simulink model "IEEE_39_case2"  (R2024b)
settings: Solver=ode3  StartTime=0  StopTime=40  FixedStep=Ts  MaxStep=1/60  RelTol=1e-3  AbsTol=1e-3  EnableMultiTasking=on
values from neighbouring files (symbols this model uses):
  c_f = c_f*Cb    [fun00_GFL_pu_2_normial.m]    (also in fun00_GFM_pu_2_normial.m)
  Dt = 0    [s02_case1.m]    (also in s02_case2.m; s03_case3.m; s03_case4.m; s03_case5.m)
  dw0_sm = 0    [s02_case1.m]    (also in s02_case2.m; s03_case3.m; s03_case4.m; s03_case5.m)
  Emax = 1.3    [s02_case1.m]    (also in s02_case2.m; s03_case3.m; s03_case4.m; s03_case5.m)
  Emin = 0.5    [s02_case1.m]    (also in s02_case2.m; s03_case3.m; s03_case4.m; s03_case5.m)
  Epss = 0.09    [s02_case1.m]    (also in s02_case2.m; s03_case3.m; s03_case4.m; s03_case5.m)
  fb = fn    (= 60)    [s02_case1.m]    (also in s02_case2.m; s03_case3.m; s03_case4.m; s03_case5.m)
  fn_sm = fn*ones(1,10)    [s02_case1.m]    (also in s02_case2.m; s03_case3.m; s03_case4.m; s03_case5.m)
  H_sm = [5,3.03,3.58,2.86,2.6,3.48,2.64,2.43,3.45,4.2]    [s02_case1.m]    (also in s02_case2.m; s03_case3.m; s03_case4.m; s03_case5.m)
  ia0_sm = 0    [s02_case1.m]    (also in s02_case2.m; s03_case3.m; s03_case4.m; s03_case5.m)
  ib0_sm = 0    [s02_case1.m]    (also in s02_case2.m; s03_case3.m; s03_case4.m; s03_case5.m)
  ic0_sm = 0    [s02_case1.m]    (also in s02_case2.m; s03_case3.m; s03_case4.m; s03_case5.m)
  Kd_sm = 0*ones(1,10)    [s02_case1.m]    (also in s02_case2.m; s03_case3.m; s03_case4.m; s03_case5.m)
  Ke = 1000    [s02_case1.m]    (also in s02_case2.m; s03_case3.m; s03_case4.m; s03_case5.m)
  ki_i = ki_i_pu*Vb_p_ph/Ib_p_ph    [fun00_GFL_pu_2_normial.m]    (also in fun00_GFM_pu_2_normial.m)
  ki_p = ki_p_pu/Sb*Ib_p_ph    [fun00_GFL_pu_2_normial.m]
  ki_pll = ki_pll/Vb_p_ph    [fun00_GFL_pu_2_normial.m]
  ki_q = ki_q_pu/Sb*Ib_p_ph    [fun00_GFL_pu_2_normial.m]
  kp_i = kp_i_pu*Vb_p_ph/Ib_p_ph    [fun00_GFL_pu_2_normial.m]    (also in fun00_GFM_pu_2_normial.m)
  kp_p = kp_p_pu/Sb*Ib_p_ph    [fun00_GFL_pu_2_normial.m]
  kp_pll = kp_pll/Vb_p_ph    [fun00_GFL_pu_2_normial.m]
  kp_q = kp_q_pu/Sb*Ib_p_ph    [fun00_GFL_pu_2_normial.m]
  Ks = 1    [s02_case1.m]    (also in s02_case2.m; s03_case3.m; s03_case4.m; s03_case5.m)
  l_f = l_f*Lb    [fun00_GFL_pu_2_normial.m]    (also in fun00_GFM_pu_2_normial.m)
  line = [     1	2	0.0035	0.0411	0.6987	0	100	345 ... (first row only)    [s02_case1.m]    (also in s02_case2.m; s03_case3.m; s03_case4.m; s03_case5.m)
  line_pu = line    [s02_case1.m]    (also in s02_case2.m; s03_case3.m; s03_case4.m; s03_case5.m)
  p = 1    [s02_case1.m]    (also in s02_case2.m; s03_case3.m; s03_case4.m; s03_case5.m)
  pha0_sm = 0    [s02_case1.m]    (also in s02_case2.m; s03_case3.m; s03_case4.m; s03_case5.m)
  phb0_sm = 0    [s02_case1.m]    (also in s02_case2.m; s03_case3.m; s03_case4.m; s03_case5.m)
  phc0_sm = 0    [s02_case1.m]    (also in s02_case2.m; s03_case3.m; s03_case4.m; s03_case5.m)
  Pn_sm = 1000*ones(1,num_gen)    [s02_case1.m]    (also in s02_case2.m; s03_case3.m; s03_case4.m; s03_case5.m)
  Pref_sm = [500 250 600 978 510 650 560 540 830 550]./Pn_sm    [s02_case1.m]    (also in s02_case2.m; s03_case3.m; s03_case4.m; s03_case5.m)
  pset = p_set_pu*Sb    [fun00_GFL_pu_2_normial.m]
  qset = q_set_pu*Sb    [fun00_GFL_pu_2_normial.m]
  R = 0.05    [s02_case1.m]    (also in s02_case2.m; s03_case3.m; s03_case4.m; s03_case5.m)
  r_f = r_f*Zb    [fun00_GFL_pu_2_normial.m]    (also in fun00_GFM_pu_2_normial.m)
  rs = 0.28    [s02_case1.m]    (also in s02_case2.m; s03_case3.m; s03_case4.m; s03_case5.m)
  Sb = 1000*10^6    (= 1000000000)    [s02_case1.m]    (also in s02_case2.m; s03_case3.m; s03_case4.m; s03_case5.m)
  T2 = 0.5    [s02_case1.m]    (also in s02_case2.m; s03_case3.m; s03_case4.m; s03_case5.m)
  T3 = 0.5    [s02_case1.m]    (also in s02_case2.m; s03_case3.m; s03_case4.m; s03_case5.m)
  t_s = 30    [s02_case1.m]    (also in s02_case2.m; s03_case3.m = 70; s03_case4.m = 70; s03_case5.m = 70)
  Te = 0.05    [s02_case1.m]    (also in s02_case2.m; s03_case3.m; s03_case4.m; s03_case5.m)
  Tfa = 3    [s02_case1.m]    (also in s02_case2.m; s03_case3.m; s03_case4.m; s03_case5.m)
  Tfb = 10    [s02_case1.m]    (also in s02_case2.m; s03_case3.m; s03_case4.m; s03_case5.m)
  theta0_sm = 0    [s02_case1.m]    (also in s02_case2.m; s03_case3.m; s03_case4.m; s03_case5.m)
  Ts = 1e-5    (= 1e-05)    [s02_case1.m]    (also in s02_case2.m; s03_case3.m; s03_case4.m; s03_case5.m)
  Ts1 = 0.76    [s02_case1.m]    (also in s02_case2.m; s03_case3.m; s03_case4.m; s03_case5.m)
  Ts2 = 0.1    [s02_case1.m]    (also in s02_case2.m; s03_case3.m; s03_case4.m; s03_case5.m)
  Ts3 = 0.76    [s02_case1.m]    (also in s02_case2.m; s03_case3.m; s03_case4.m; s03_case5.m)
  Ts4 = 0.1    [s02_case1.m]    (also in s02_case2.m; s03_case3.m; s03_case4.m; s03_case5.m)
  Ts5 = 10    [s02_case1.m]    (also in s02_case2.m; s03_case3.m; s03_case4.m; s03_case5.m)
  Un_sm = [345,22,22,22,22,22,22,22,345,22]    [s02_case1.m]    (also in s02_case2.m; s03_case3.m; s03_case4.m; s03_case5.m)
  Vb_gfm = 22*10^3    (= 22000)    [s02_case1.m]    (also in s02_case2.m; s03_case3.m; s03_case4.m; s03_case5.m)
  Vdc = 3*Vb_p_ph    [fun00_GFL_pu_2_normial.m]    (also in fun00_GFM_pu_2_normial.m)
  Vmax = 2    [s02_case1.m]    (also in s02_case2.m; s03_case3.m; s03_case4.m; s03_case5.m)
  Vmin = 0    [s02_case1.m]    (also in s02_case2.m; s03_case3.m; s03_case4.m; s03_case5.m)
  Vref_sm = 1*ones(1,10)    [s02_case1.m]    (also in s02_case2.m; s03_case3.m; s03_case4.m; s03_case5.m)
  w_b = fb*2*pi    [fun00_GFL_pu_2_normial.m]    (also in fun00_GFM_pu_2_normial.m; s02_case1.m = 376.991118431; s02_case2.m = 376.991118431; s03_case3.m = 376.991118431)
  wb = w_b    (= 376.991118431)    [s02_case1.m]    (also in s02_case2.m; s03_case3.m; s03_case4.m; s03_case5.m)
  xd = xd_t    (= 0.296)    [s02_case1.m]    (also in s02_case2.m; s03_case3.m; s03_case4.m; s03_case5.m)
undefined symbols (not defined in the file or in its folder): c_f_gfm, D1, D_p_gfm, D_q_gfm, Delta, DiscIntNeverNeededParam, Init, Init_GFL, J_gfm, Ka, Kf, ki_i_gfm, ki_pll_s, ki_vc_gfm, kp_i_gfm, kp_pll_s, kp_vc_gfm, l_f_gfm, P_set_gfm, Q_set_gfm, r_f_gfm, Ta, Tf, Vb, Vdc_gfm
libraries: spsThreePhaseVIMeasurementLib x76, spsabctodq0Lib x53, spsThreePhaseSeriesRLCBranchLib x52, slpidlib x50, spsThreePhaseParallelRLCLoadLib x20, spsThreePhaseTransformerTwoWindingsLib x12, spsdq0toabcLib x9, spsGroundLib x9, spsPowerPositiveSequenceLib x9, spsUniversalBridgeLib x9, spsDCVoltageSourceLib x9, spsFirstOrderFilterLib x1
(part 2 of 10)

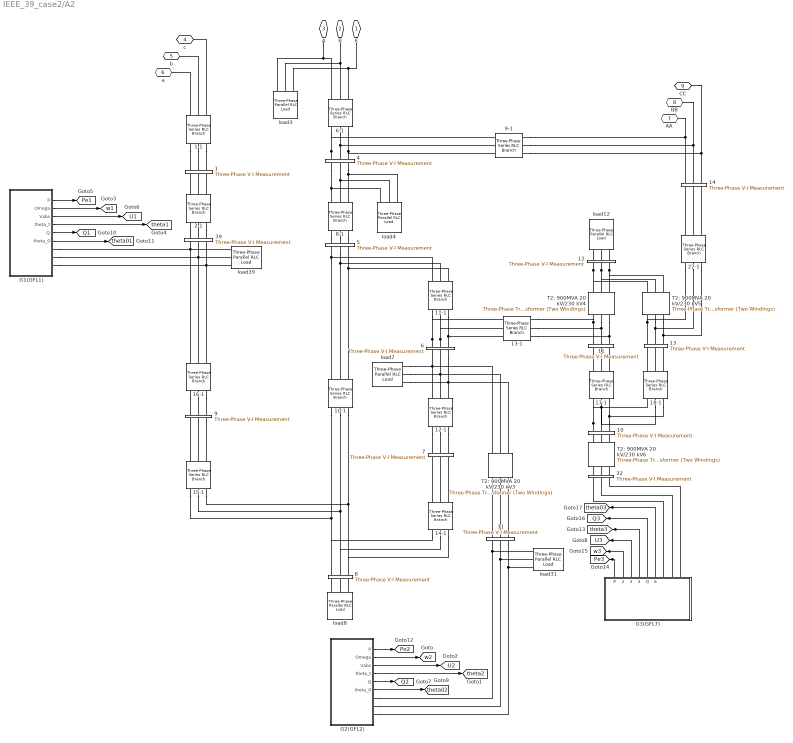
== system IEEE_39_case2/A2 ==
  1 : spsThreePhaseVIMeasurementLib/Three-Phase V-I Measurement  VoltageMeasurement=phase-to-phase  SetLabelV=on  LabelV=Vabc_1  Vpu=off  VpuLL=on  CurrentMeasurement=no  SetLabelI=on  LabelI=Iabc_B2  Ipu=off  Pbase=100e6  Vbase=Bus(1,2)*1e3  OutputType=Complex  PhasorSimulation=off  PSBequivalent=0
  1-1 : spsThreePhaseSeriesRLCBranchLib/Three-Phase Series RLC Branch  LConnTagsString=A|B|C  RConnTagsString=A|B|C  BranchType=RL  Resistance=line(1,3)  Inductance=line(1,4)  Capacitance=1e-6  Measurements=None
  10 : spsThreePhaseVIMeasurementLib/Three-Phase V-I Measurement  VoltageMeasurement=phase-to-phase  SetLabelV=on  LabelV=Vabc_10  Vpu=off  VpuLL=on  CurrentMeasurement=no  SetLabelI=on  LabelI=Iabc_B2  Ipu=off  Pbase=100e6  Vbase=Bus(10,2)*1e3  OutputType=Complex  PhasorSimulation=off  PSBequivalent=0
  10-1 : spsThreePhaseSeriesRLCBranchLib/Three-Phase Series RLC Branch  LConnTagsString=A|B|C  RConnTagsString=A|B|C  BranchType=RL  Resistance=line(10,3)  Inductance=line(10,4)  Capacitance=1e-6  Measurements=None
  11 : spsThreePhaseVIMeasurementLib/Three-Phase V-I Measurement  VoltageMeasurement=phase-to-phase  SetLabelV=on  LabelV=Vabc_11  Vpu=off  VpuLL=on  CurrentMeasurement=no  SetLabelI=on  LabelI=Iabc_B2  Ipu=off  Pbase=100e6  Vbase=Bus(11,2)*1e3  OutputType=Complex  PhasorSimulation=off  PSBequivalent=0
  11-1 : spsThreePhaseSeriesRLCBranchLib/Three-Phase Series RLC Branch  LConnTagsString=A|B|C  RConnTagsString=A|B|C  BranchType=RL  Resistance=line(11,3)  Inductance=line(11,4)  Capacitance=1e-6  Measurements=None
  12 : spsThreePhaseVIMeasurementLib/Three-Phase V-I Measurement  VoltageMeasurement=phase-to-phase  SetLabelV=on  LabelV=Vabc_12  Vpu=off  VpuLL=on  CurrentMeasurement=no  SetLabelI=on  LabelI=Iabc_B2  Ipu=off  Pbase=100e6  Vbase=Bus(12,2)*1e3  OutputType=Complex  PhasorSimulation=off  PSBequivalent=0
  12-1 : spsThreePhaseSeriesRLCBranchLib/Three-Phase Series RLC Branch  LConnTagsString=A|B|C  RConnTagsString=A|B|C  BranchType=RL  Resistance=line(12,3)  Inductance=line(12,4)  Capacitance=1e-6  Measurements=None
  13 : spsThreePhaseVIMeasurementLib/Three-Phase V-I Measurement  VoltageMeasurement=phase-to-phase  SetLabelV=on  LabelV=Vabc_13  Vpu=off  VpuLL=on  CurrentMeasurement=no  SetLabelI=on  LabelI=Iabc_B2  Ipu=off  Pbase=100e6  Vbase=Bus(13,2)*1e3  OutputType=Complex  PhasorSimulation=off  PSBequivalent=0
  13-1 : spsThreePhaseSeriesRLCBranchLib/Three-Phase Series RLC Branch  LConnTagsString=A|B|C  RConnTagsString=A|B|C  BranchType=RL  Resistance=line(13,3)  Inductance=line(13,4)  Capacitance=1e-6  Measurements=None
  14 : spsThreePhaseVIMeasurementLib/Three-Phase V-I Measurement  VoltageMeasurement=phase-to-phase  SetLabelV=on  LabelV=Vabc_14  Vpu=off  VpuLL=on  CurrentMeasurement=no  SetLabelI=on  LabelI=Iabc_B2  Ipu=off  Pbase=100e6  Vbase=Bus(14,2)*1e3  OutputType=Complex  PhasorSimulation=off  PSBequivalent=0
  14-1 : spsThreePhaseSeriesRLCBranchLib/Three-Phase Series RLC Branch  LConnTagsString=A|B|C  RConnTagsString=A|B|C  BranchType=RL  Resistance=line(14,3)  Inductance=line(14,4)  Capacitance=1e-6  Measurements=None
  15-1 : spsThreePhaseSeriesRLCBranchLib/Three-Phase Series RLC Branch  LConnTagsString=A|B|C  RConnTagsString=A|B|C  BranchType=RL  Resistance=line(15,3)  Inductance=line(15,4)  Capacitance=1e-6  Measurements=None
  16-1 : spsThreePhaseSeriesRLCBranchLib/Three-Phase Series RLC Branch  LConnTagsString=A|B|C  RConnTagsString=A|B|C  BranchType=RL  Resistance=line(16,3)  Inductance=line(16,4)  Capacitance=1e-6  Measurements=None
  17-1 : spsThreePhaseSeriesRLCBranchLib/Three-Phase Series RLC Branch  LConnTagsString=A|B|C  RConnTagsString=A|B|C  BranchType=RL  Resistance=line(17,3)  Inductance=line(17,4)  Capacitance=1e-6  Measurements=None
  18-1 : spsThreePhaseSeriesRLCBranchLib/Three-Phase Series RLC Branch  LConnTagsString=A|B|C  RConnTagsString=A|B|C  BranchType=RL  Resistance=line(18,3)  Inductance=line(18,4)  Capacitance=1e-6  Measurements=None
  2-1 : spsThreePhaseSeriesRLCBranchLib/Three-Phase Series RLC Branch  LConnTagsString=A|B|C  RConnTagsString=A|B|C  BranchType=RL  Resistance=line(2,3)  Inductance=line(2,4)  Capacitance=1e-6  Measurements=None
  22-1 : spsThreePhaseSeriesRLCBranchLib/Three-Phase Series RLC Branch  LConnTagsString=A|B|C  RConnTagsString=A|B|C  BranchType=RL  Resistance=line(22,3)  Inductance=line(22,4)  Capacitance=1e-6  Measurements=None
  31 : spsThreePhaseVIMeasurementLib/Three-Phase V-I Measurement  VoltageMeasurement=phase-to-phase  SetLabelV=on  LabelV=Vabc_31  Vpu=off  VpuLL=on  CurrentMeasurement=no  SetLabelI=on  LabelI=Iabc_B2  Ipu=off  Pbase=100e6  Vbase=Bus(31,2)*1e3  OutputType=Complex  PhasorSimulation=off  PSBequivalent=0
  32 : spsThreePhaseVIMeasurementLib/Three-Phase V-I Measurement  VoltageMeasurement=phase-to-phase  SetLabelV=on  LabelV=Vabc_32  Vpu=off  VpuLL=off  CurrentMeasurement=yes  SetLabelI=on  LabelI=Iabc_32  Ipu=off  Pbase=100e6  Vbase=Bus(32,2)*1e3  OutputType=Complex  PhasorSimulation=off  PSBequivalent=0
  39 : spsThreePhaseVIMeasurementLib/Three-Phase V-I Measurement  VoltageMeasurement=phase-to-phase  SetLabelV=on  LabelV=Vabc_39  Vpu=off  VpuLL=on  CurrentMeasurement=no  SetLabelI=on  LabelI=Iabc_B2  Ipu=off  Pbase=100e6  Vbase=Bus(39,2)*1e3  OutputType=Complex  PhasorSimulation=off  PSBequivalent=0
  4 : spsThreePhaseVIMeasurementLib/Three-Phase V-I Measurement  VoltageMeasurement=phase-to-phase  SetLabelV=on  LabelV=Vabc_B4  Vpu=off  VpuLL=on  CurrentMeasurement=yes  SetLabelI=on  LabelI=Iabc_B4  Ipu=off  Pbase=100e6  Vbase=Bus(4,2)*1e3  OutputType=Complex  PhasorSimulation=off  PSBequivalent=0
  5 : spsThreePhaseVIMeasurementLib/Three-Phase V-I Measurement  VoltageMeasurement=phase-to-phase  SetLabelV=on  LabelV=Vabc_5  Vpu=off  VpuLL=on  CurrentMeasurement=no  SetLabelI=on  LabelI=Iabc_B2  Ipu=off  Pbase=100e6  Vbase=Bus(5,2)*1e3  OutputType=Complex  PhasorSimulation=off  PSBequivalent=0
  6 : spsThreePhaseVIMeasurementLib/Three-Phase V-I Measurement  VoltageMeasurement=phase-to-phase  SetLabelV=on  LabelV=Vabc_6  Vpu=off  VpuLL=on  CurrentMeasurement=no  SetLabelI=on  LabelI=Iabc_B2  Ipu=off  Pbase=100e6  Vbase=Bus(6,2)*1e3  OutputType=Complex  PhasorSimulation=off  PSBequivalent=0
  6-1 : spsThreePhaseSeriesRLCBranchLib/Three-Phase Series RLC Branch  LConnTagsString=A|B|C  RConnTagsString=A|B|C  BranchType=RL  Resistance=line(6,3)  Inductance=line(6,4)  Capacitance=1e-6  Measurements=None
  7 : spsThreePhaseVIMeasurementLib/Three-Phase V-I Measurement  VoltageMeasurement=phase-to-phase  SetLabelV=on  LabelV=Vabc_7  Vpu=off  VpuLL=on  CurrentMeasurement=no  SetLabelI=on  LabelI=Iabc_B2  Ipu=off  Pbase=100e6  Vbase=Bus(8,2)*1e3  OutputType=Complex  PhasorSimulation=off  PSBequivalent=0
  8 : spsThreePhaseVIMeasurementLib/Three-Phase V-I Measurement  VoltageMeasurement=phase-to-phase  SetLabelV=on  LabelV=Vabc_8  Vpu=off  VpuLL=on  CurrentMeasurement=no  SetLabelI=on  LabelI=Iabc_B2  Ipu=off  Pbase=100e6  Vbase=Bus(8,2)*1e3  OutputType=Complex  PhasorSimulation=off  PSBequivalent=0
  8-1 : spsThreePhaseSeriesRLCBranchLib/Three-Phase Series RLC Branch  LConnTagsString=A|B|C  RConnTagsString=A|B|C  BranchType=RL  Resistance=line(8,3)  Inductance=line(8,4)  Capacitance=1e-6  Measurements=None
  9 : spsThreePhaseVIMeasurementLib/Three-Phase V-I Measurement  VoltageMeasurement=phase-to-phase  SetLabelV=on  LabelV=Vabc_9  Vpu=off  VpuLL=on  CurrentMeasurement=no  SetLabelI=on  LabelI=Iabc_B2  Ipu=off  Pbase=100e6  Vbase=Bus(9,2)*1e3  OutputType=Complex  PhasorSimulation=off  PSBequivalent=0
  9-1 : spsThreePhaseSeriesRLCBranchLib/Three-Phase Series RLC Branch  LConnTagsString=A|B|C  RConnTagsString=A|B|C  BranchType=RL  Resistance=line(9,3)  Inductance=line(9,4)  Capacitance=1e-6  Measurements=None
  G1(GFL1) : Subsystem  mask{Pnom=Sb, Vnom=Vb(1), Fnom=fb, Vdc_nom=Vdc(1), RLC_Filter=[r_f(1) l_f(1) c_f(1)], Pref=pset(1), Qref=qset(1), PLL_p=kp_pll(1), PLL_i=ki_pll(1), Voltage_P=kp_q(1), Voltage_I=ki_q(1), Current_P=kp_i(1), Current_I=ki_i(1), Power_P=kp_p(1), Power_I=ki_p(1), kf=1, InitialV=Init_GFL(1)}
      mask prompts: Pnom "Rated Power(VA)"; Vnom "Rated L-L RMS Voltage(V)"; Fnom "Rated Frequency(Hz)"; Vdc_nom "DC capacitor voltage(V)"; RLC_Filter "Grid-side coupling impedance(p.u.)"; Pref "Active Power Setting"; Qref "Reactive Power Setting"; PLL_p "PL Proportional Gain"; PLL_i "PLL Integral Gain"; Voltage_P "Voltage Proportional Gain"; Voltage_I "Voltage Integral Gain"; Current_P "Current Proportional Gain"; Current_I "Current Integral Gain"; Power_P "Power Proportional Gain"; Power_I "Power Integral Gain"; kf "Feedforward Gain"; InitialV "Initial Condition"
      mask init:
      | R_f=RLC_Filter(1);
      | L_f=RLC_Filter(2);
      | C_f=RLC_Filter(3);
      mask Display: disp('GFL');
  G2(GFL2) : Subsystem  mask{Pnom=Sb, Vnom=Vb(2), Fnom=fb, Vdc_nom=Vdc(2), RLC_Filter=[r_f(2) l_f(2) c_f(2)], Pref=pset(2), Qref=qset(2), PLL_p=kp_pll(2), PLL_i=ki_pll(2), Voltage_P=kp_q(2), Voltage_I=ki_q(2), Current_P=kp_i(2), Current_I=ki_i(2), Power_P=kp_p(2), Power_I=ki_p(2), kf=1, InitialV=Init_GFL(2)}
      mask prompts: Pnom "Rated Power(VA)"; Vnom "Rated L-L RMS Voltage(V)"; Fnom "Rated Frequency(Hz)"; Vdc_nom "DC capacitor voltage(V)"; RLC_Filter "Grid-side coupling impedance(p.u.)"; Pref "Active Power Setting"; Qref "Reactive Power Setting"; PLL_p "PL Proportional Gain"; PLL_i "PLL Integral Gain"; Voltage_P "Voltage Proportional Gain"; Voltage_I "Voltage Integral Gain"; Current_P "Current Proportional Gain"; Current_I "Current Integral Gain"; Power_P "Power Proportional Gain"; Power_I "Power Integral Gain"; kf "Feedforward Gain"; InitialV "Initial Condition"
      mask init:
      | R_f=RLC_Filter(1);
      | L_f=RLC_Filter(2);
      | C_f=RLC_Filter(3);
      mask Display: disp('GFL');
  G3(GFL7) : Subsystem  mask{Pnom=Sb, Vnom=Vb(7), Fnom=fb, Vdc_nom=Vdc(7), RLC_Filter=[r_f(7) l_f(7) c_f(7)], Pref=pset(7), Qref=qset(7), PLL_p=kp_pll(7), PLL_i=ki_pll(7), Voltage_P=kp_q(7), Voltage_I=ki_q(7), Current_P=kp_i(7), Current_I=ki_i(7), Power_P=kp_p(7), Power_I=ki_p(7), kf=1, InitialV=Init_GFL(7)}
      mask prompts: Pnom "Rated Power(VA)"; Vnom "Rated L-L RMS Voltage(V)"; Fnom "Rated Frequency(Hz)"; Vdc_nom "DC capacitor voltage(V)"; RLC_Filter "Grid-side coupling impedance(p.u.)"; Pref "Active Power Setting"; Qref "Reactive Power Setting"; PLL_p "PL Proportional Gain"; PLL_i "PLL Integral Gain"; Voltage_P "Voltage Proportional Gain"; Voltage_I "Voltage Integral Gain"; Current_P "Current Proportional Gain"; Current_I "Current Integral Gain"; Power_P "Power Proportional Gain"; Power_I "Power Integral Gain"; kf "Feedforward Gain"; InitialV "Initial Condition"
      mask init:
      | R_f=RLC_Filter(1);
      | L_f=RLC_Filter(2);
      | C_f=RLC_Filter(3);
      mask Display: disp('GFL');
  T2: 900MVA 20 kV/230 kV3 : spsThreePhaseTransformerTwoWindingsLib/Three-Phase Transformer (Two Windings)  Winding1Connection=Delta (D1)  Winding2Connection=Yg  CoreType=Three single-phase transformers  SetSaturation=off  Hysteresis=off  DataFile='hysteresis'  SetInitialFlux=off  Measurements=None  UNITS=pu  NominalPower=[ 100e6 60 ]  Winding1="[ 22e3*1.0 1e-6  0]"  Winding2="[ 345e3*1.0  1e-6  line_pu(end,4) ]"  Rm=500  Lm=500  L0=0.5  Saturation="[ 0,0  ;  0.005,1.2  ;  1.0,1.4 ]"  InitialFluxes=[ 0.8 , -0.8 , 0.7 ]  BreakLoop=off  DiscreteSolver=Trapezoidal iterative  DataType=off  TransfoNumber=0
  T2: 900MVA 20 kV/230 kV4 : spsThreePhaseTransformerTwoWindingsLib/Three-Phase Transformer (Two Windings)  Winding1Connection=Y  Winding2Connection=Y  CoreType=Three single-phase transformers  SetSaturation=off  Hysteresis=off  DataFile='hysteresis'  SetInitialFlux=off  Measurements=None  UNITS=pu  NominalPower=[ 100e6 60 ]  Winding1="[ 345e3 .0008  0]"  Winding2="[ 230e3*1.00  .0008  0.0435]"  Rm=500  Lm=500  L0=0.5  Saturation="[ 0,0  ;  0.005,1.2  ;  1.0,1.4 ]"  InitialFluxes=[ 0.8 , -0.8 , 0.7 ]  BreakLoop=off  DiscreteSolver=Trapezoidal iterative  DataType=off  TransfoNumber=0
  T2: 900MVA 20 kV/230 kV5 : spsThreePhaseTransformerTwoWindingsLib/Three-Phase Transformer (Two Windings)  Winding1Connection=Y  Winding2Connection=Y  CoreType=Three single-phase transformers  SetSaturation=off  Hysteresis=off  DataFile='hysteresis'  SetInitialFlux=off  Measurements=None  UNITS=pu  NominalPower=[ 100e6 60 ]  Winding1="[ 345e3 0.0008  0]"  Winding2="[ 230e3*1.00 0.0008  0.0435]"  Rm=500  Lm=500  L0=0.5  Saturation="[ 0,0  ;  0.005,1.2  ;  1.0,1.4 ]"  InitialFluxes=[ 0.8 , -0.8 , 0.7 ]  BreakLoop=off  DiscreteSolver=Trapezoidal iterative  DataType=off  TransfoNumber=0
  T2: 900MVA 20 kV/230 kV6 : spsThreePhaseTransformerTwoWindingsLib/Three-Phase Transformer (Two Windings)  Winding1Connection=Delta (D1)  Winding2Connection=Yg  CoreType=Three single-phase transformers  SetSaturation=off  Hysteresis=off  DataFile='hysteresis'  SetInitialFlux=off  Measurements=None  UNITS=pu  NominalPower=[ 100e6 60 ]  Winding1="[ 22e3*1.0 1e-6  0]"  Winding2="[ 345e3*1.0   1e-6    line_pu(19,4) ]"  Rm=500  Lm=500  L0=0.5  Saturation="[ 0,0  ;  0.005,1.2  ;  1.0,1.4 ]"  InitialFluxes=[ 0.8 , -0.8 , 0.7 ]  BreakLoop=off  DiscreteSolver=Trapezoidal iterative  DataType=off  TransfoNumber=0
  load12 : spsThreePhaseParallelRLCLoadLib/Three-Phase Parallel RLC Load  LConnTagsString=A|B|C  Configuration=Y (grounded)  NominalVoltage=(230000)*0.939625  Vabc=[1e3 1e3 1e3]  Vabcp=[1e3 1e3 1e3]  NominalFrequency=60  UnbalancedPower=off  ActivePower=7.5e6  InductivePower=88e6  CapacitivePower=0  Pabc=[10e3 9e3 11e3]  QLabc=[100 90 110]  QCabc=[100 90 110]  Pabcp=[10e3 9e3 11e3]  QLabcp=[100 90 110]  QCabcp=[100 90 110]  Measurements=None  LoadType=constant PQ
  load3 : spsThreePhaseParallelRLCLoadLib/Three-Phase Parallel RLC Load  LConnTagsString=A|B|C  Configuration=Y (grounded)  NominalVoltage=(345000)*0.992094  Vabc=[1e3 1e3 1e3]  Vabcp=[1e3 1e3 1e3]  NominalFrequency=60  UnbalancedPower=off  ActivePower=322e6  InductivePower=2.4e6  CapacitivePower=0  Pabc=[10e3 9e3 11e3]  QLabc=[100 90 110]  QCabc=[100 90 110]  Pabcp=[10e3 9e3 11e3]  QLabcp=[100 90 110]  QCabcp=[100 90 110]  Measurements=None  LoadType=constant PQ
  load31 : spsThreePhaseParallelRLCLoadLib/Three-Phase Parallel RLC Load  LConnTagsString=A|B|C  Configuration=Y (grounded)  NominalVoltage=(22000)*0.982  Vabc=[1e3 1e3 1e3]  Vabcp=[1e3 1e3 1e3]  NominalFrequency=60  UnbalancedPower=off  ActivePower=9.2e6  InductivePower=4.6e6  CapacitivePower=0  Pabc=[10e3 9e3 11e3]  QLabc=[100 90 110]  QCabc=[100 90 110]  Pabcp=[10e3 9e3 11e3]  QLabcp=[100 90 110]  QCabcp=[100 90 110]  Measurements=None  LoadType=constant PQ
  load39 : spsThreePhaseParallelRLCLoadLib/Three-Phase Parallel RLC Load  LConnTagsString=A|B|C  Configuration=Y (grounded)  NominalVoltage=(345000)*1.03  Vabc=[1e3 1e3 1e3]  Vabcp=[1e3 1e3 1e3]  NominalFrequency=60  UnbalancedPower=off  ActivePower=1104e6  InductivePower=250e6  CapacitivePower=0  Pabc=[10e3 9e3 11e3]  QLabc=[100 90 110]  QCabc=[100 90 110]  Pabcp=[10e3 9e3 11e3]  QLabcp=[100 90 110]  QCabcp=[100 90 110]  Measurements=None  LoadType=constant PQ
  load4 : spsThreePhaseParallelRLCLoadLib/Three-Phase Parallel RLC Load  LConnTagsString=A|B|C  Configuration=Y (grounded)  NominalVoltage=(345000)*0.95637  Vabc=[1e3 1e3 1e3]  Vabcp=[1e3 1e3 1e3]  NominalFrequency=60  UnbalancedPower=off  ActivePower=500e6  InductivePower=184e6  CapacitivePower=0  Pabc=[10e3 9e3 11e3]  QLabc=[100 90 110]  QCabc=[100 90 110]  Pabcp=[10e3 9e3 11e3]  QLabcp=[100 90 110]  QCabcp=[100 90 110]  Measurements=None  LoadType=constant PQ
  load7 : spsThreePhaseParallelRLCLoadLib/Three-Phase Parallel RLC Load  LConnTagsString=A|B|C  Configuration=Y (grounded)  NominalVoltage=(345000)*0.956463  Vabc=[1e3 1e3 1e3]  Vabcp=[1e3 1e3 1e3]  NominalFrequency=60  UnbalancedPower=off  ActivePower=233.8e6  InductivePower=84e6  CapacitivePower=0  Pabc=[10e3 9e3 11e3]  QLabc=[100 90 110]  QCabc=[100 90 110]  Pabcp=[10e3 9e3 11e3]  QLabcp=[100 90 110]  QCabcp=[100 90 110]  Measurements=None  LoadType=constant PQ
  load8 : spsThreePhaseParallelRLCLoadLib/Three-Phase Parallel RLC Load  LConnTagsString=A|B|C  Configuration=Y (grounded)  NominalVoltage=(345000)*0.954036  Vabc=[1e3 1e3 1e3]  Vabcp=[1e3 1e3 1e3]  NominalFrequency=60  UnbalancedPower=off  ActivePower=522e6  InductivePower=176e6  CapacitivePower=0  Pabc=[10e3 9e3 11e3]  QLabc=[100 90 110]  QCabc=[100 90 110]  Pabcp=[10e3 9e3 11e3]  QLabcp=[100 90 110]  QCabcp=[100 90 110]  Measurements=None  LoadType=constant PQ
  C : PMIOPort  Side=Left
  B : PMIOPort  Port=2  Side=Left
  A : PMIOPort  Port=3  Side=Left
  c : PMIOPort  Port=4  Side=Left
  b : PMIOPort  Port=5  Side=Left
  a : PMIOPort  Port=6  Side=Left
  AA : PMIOPort  Port=7  Side=Right
  BB : PMIOPort  Port=8  Side=Right
  CC : PMIOPort  Port=9  Side=Right
  tag scope: Pe1=global, Pe2=global, Pe3=global, Q1=global, Q2=global, Q3=global, U1=global, U2=global, U3=global, theta01=global, theta02=global, theta03=global, theta1=global, theta2=global, theta3=global, w1=global, w2=global, w3=global
  wires:
  G2(GFL2)/1(P) -> [Pe2]
  G2(GFL2)/4(theta_t) -> [theta2]
  G2(GFL2)/2(Omega) -> [w2]
  G2(GFL2)/3(Vabs) -> [U2]
  G1(GFL1)/4(theta_t) -> [theta1]
  G1(GFL1)/3(Vabs) -> [U1]
  G1(GFL1)/2(Omega) -> [w1]
  G1(GFL1)/1(P) -> [Pe1]
  G2(GFL2)/5(Q) -> [Q2]
  G2(GFL2)/6(theta_0) -> [theta02]
  G1(GFL1)/5(Q) -> [Q1]
  G1(GFL1)/6(theta_0) -> [theta01]
  G3(GFL7)/1(P) -> [Pe3]
  G3(GFL7)/2(Omega) -> [w3]
  G3(GFL7)/3(Vabs) -> [U3]
  G3(GFL7)/4(theta_t) -> [theta3]
  G3(GFL7)/6(theta_0) -> [theta03]
  G3(GFL7)/5(Q) -> [Q3]
  connections:
  load3/LConn3 -- 6-1/LConn3 -- C/RConn1
  17-1/LConn1 -- 11/RConn1
  5/RConn2 -- 10-1/LConn2 -- 11-1/LConn2
  14-1/LConn1 -- 7/LConn1
  14-1/RConn3 -- 8/LConn3 -- 10-1/RConn3 -- 15-1/RConn3
  load8/LConn1 -- 8/RConn1
  14-1/LConn2 -- 7/LConn2
  18-1/LConn2 -- 13/RConn2
  2-1/LConn2 -- 1/RConn2
  14-1/RConn2 -- 8/LConn2 -- 10-1/RConn2 -- 15-1/RConn2
  T2: 900MVA 20 kV/230 kV6/RConn1 -- 10/RConn1
  9-1/LConn3 -- CC/RConn1 -- 14/RConn3
  1-1/RConn1 -- 1/LConn1
  12-1/LConn1 -- T2: 900MVA 20 kV/230 kV3/RConn1 -- load7/LConn1 -- 6/RConn1
  2-1/LConn3 -- 1/RConn3
  12/RConn1 -- T2: 900MVA 20 kV/230 kV5/RConn1 -- T2: 900MVA 20 kV/230 kV4/RConn1
  12-1/RConn1 -- 7/RConn1
  39/RConn1 -- G1(GFL1)/RConn1 -- 16-1/LConn1 -- load39/LConn1
  load31/LConn3 -- G2(GFL2)/RConn3 -- 31/RConn3
  13-1/RConn2 -- T2: 900MVA 20 kV/230 kV4/LConn2 -- 11/LConn2
  8/LConn1 -- 14-1/RConn1 -- 10-1/RConn1 -- 15-1/RConn1
  15-1/LConn3 -- 9/RConn3
  1-1/RConn3 -- 1/LConn3
  12/RConn3 -- T2: 900MVA 20 kV/230 kV5/RConn3 -- T2: 900MVA 20 kV/230 kV4/RConn3
  6/LConn1 -- 13-1/LConn1 -- 11-1/RConn1
  17-1/RConn3 -- 18-1/RConn3 -- 10/LConn3
  6/RConn3 -- T2: 900MVA 20 kV/230 kV3/RConn3 -- 12-1/LConn3 -- load7/LConn3
  6/LConn2 -- 13-1/LConn2 -- 11-1/RConn2
  9-1/LConn1 -- AA/RConn1 -- 14/RConn1
  17-1/LConn3 -- 11/RConn3
  load3/LConn2 -- B/RConn1 -- 6-1/LConn2
  2-1/RConn2 -- 39/LConn2
  13/LConn1 -- 22-1/RConn1 -- T2: 900MVA 20 kV/230 kV5/LConn1
  22-1/LConn3 -- 14/LConn3
  18-1/LConn1 -- 13/RConn1
  22-1/RConn3 -- T2: 900MVA 20 kV/230 kV5/LConn3 -- 13/LConn3
  18-1/LConn3 -- 13/RConn3
  13/LConn2 -- T2: 900MVA 20 kV/230 kV5/LConn2 -- 22-1/RConn2
  2-1/RConn1 -- 39/LConn1
  22-1/LConn2 -- 14/LConn2
  9-1/RConn2 -- 6-1/RConn2 -- 4/LConn2
  17-1/LConn2 -- 11/RConn2
  10/LConn1 -- 17-1/RConn1 -- 18-1/RConn1
  15-1/LConn2 -- 9/RConn2
  15-1/LConn1 -- 9/RConn1
  22-1/LConn1 -- 14/LConn1
  load3/LConn1 -- 6-1/LConn1 -- A/RConn1
  6-1/RConn3 -- 9-1/RConn3 -- 4/LConn3
  1-1/LConn2 -- b/RConn1
  4/LConn1 -- 9-1/RConn1 -- 6-1/RConn1
  17-1/RConn2 -- 18-1/RConn2 -- 10/LConn2
  T2: 900MVA 20 kV/230 kV3/LConn2 -- 31/LConn2
  2-1/RConn3 -- 39/LConn3
  T2: 900MVA 20 kV/230 kV6/LConn1 -- 32/LConn1
  9-1/LConn2 -- BB/RConn1 -- 14/RConn2
  1-1/RConn2 -- 1/LConn2
  10-1/LConn1 -- 11-1/LConn1 -- 5/RConn1
  2-1/LConn1 -- 1/RConn1
  16-1/RConn1 -- 9/LConn1
  14-1/LConn3 -- 7/LConn3
  4/RConn1 -- 8-1/LConn1 -- load4/LConn1
  10-1/LConn3 -- 11-1/LConn3 -- 5/RConn3
  12-1/LConn2 -- T2: 900MVA 20 kV/230 kV3/RConn2 -- load7/LConn2 -- 6/RConn2
  load31/LConn2 -- G2(GFL2)/RConn2 -- 31/RConn2
  T2: 900MVA 20 kV/230 kV6/LConn2 -- 32/LConn2
  12-1/RConn2 -- 7/RConn2
  8-1/RConn1 -- 5/LConn1
  load4/LConn2 -- 8-1/LConn2 -- 4/RConn2
  16-1/RConn3 -- 9/LConn3
  16-1/RConn2 -- 9/LConn2
  load31/LConn1 -- G2(GFL2)/RConn1 -- 31/RConn1
  4/RConn3 -- 8-1/LConn3 -- load4/LConn3
  8-1/RConn3 -- 5/LConn3
  8-1/RConn2 -- 5/LConn2
  11-1/RConn3 -- 13-1/LConn3 -- 6/LConn3
  13-1/RConn3 -- T2: 900MVA 20 kV/230 kV4/LConn3 -- 11/LConn3
  12/LConn2 -- load12/LConn2
  12/LConn3 -- load12/LConn3
  T2: 900MVA 20 kV/230 kV3/LConn1 -- 31/LConn1
  8/RConn2 -- load8/LConn2
  load8/LConn3 -- 8/RConn3
  T2: 900MVA 20 kV/230 kV6/LConn3 -- 32/LConn3
  12-1/RConn3 -- 7/RConn3
  12/RConn2 -- T2: 900MVA 20 kV/230 kV5/RConn2 -- T2: 900MVA 20 kV/230 kV4/RConn2
  T2: 900MVA 20 kV/230 kV3/LConn3 -- 31/LConn3
  T2: 900MVA 20 kV/230 kV6/RConn3 -- 10/RConn3
  T2: 900MVA 20 kV/230 kV6/RConn2 -- 10/RConn2
  13-1/RConn1 -- T2: 900MVA 20 kV/230 kV4/LConn1 -- 11/LConn1
  12/LConn1 -- load12/LConn1
  1-1/LConn3 -- c/RConn1
  1-1/LConn1 -- a/RConn1
  16-1/LConn2 -- G1(GFL1)/RConn2 -- load39/LConn2 -- 39/RConn2
  16-1/LConn3 -- G1(GFL1)/RConn3 -- load39/LConn3 -- 39/RConn3
  G3(GFL7)/RConn1 -- 32/RConn1
  G3(GFL7)/RConn2 -- 32/RConn2
  G3(GFL7)/RConn3 -- 32/RConn3

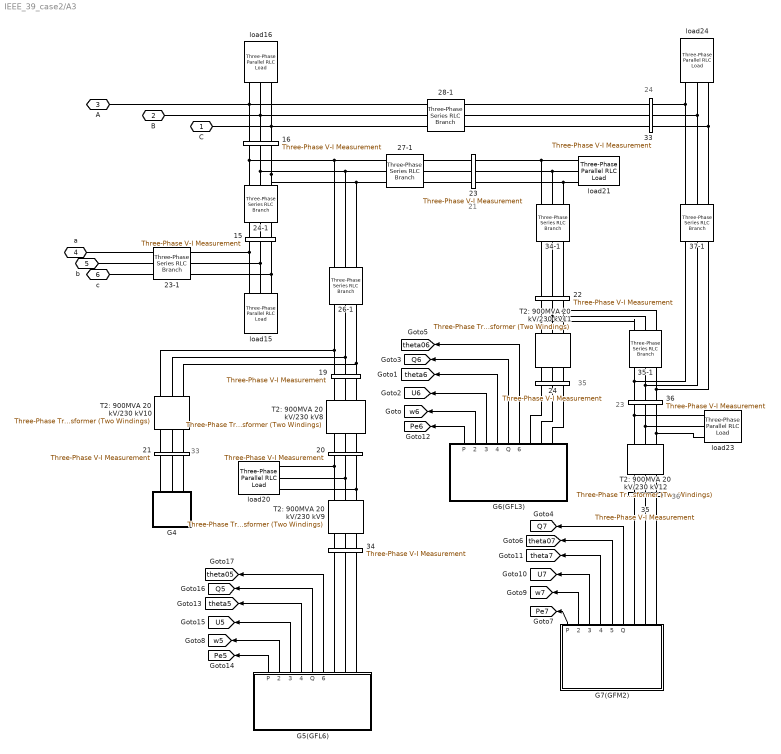
== system IEEE_39_case2/A3 ==
  note: 35
  note: 33
  note: 21
  note: 24
  note: 36
  note: 23
  15 : spsThreePhaseVIMeasurementLib/Three-Phase V-I Measurement  VoltageMeasurement=phase-to-phase  SetLabelV=on  LabelV=Vabc_15  Vpu=off  VpuLL=on  CurrentMeasurement=no  SetLabelI=on  LabelI=Iabc_B2  Ipu=off  Pbase=100e6  Vbase=Bus(15,2)*1e3  OutputType=Complex  PhasorSimulation=off  PSBequivalent=0
  16 : spsThreePhaseVIMeasurementLib/Three-Phase V-I Measurement  VoltageMeasurement=phase-to-phase  SetLabelV=on  LabelV=Vabc_16  Vpu=off  VpuLL=on  CurrentMeasurement=no  SetLabelI=on  LabelI=Iabc_B2  Ipu=off  Pbase=100e6  Vbase=Bus(16,2)*1e3  OutputType=Complex  PhasorSimulation=off  PSBequivalent=0
  19 : spsThreePhaseVIMeasurementLib/Three-Phase V-I Measurement  VoltageMeasurement=phase-to-phase  SetLabelV=on  LabelV=Vabc_19  Vpu=off  VpuLL=on  CurrentMeasurement=no  SetLabelI=on  LabelI=Iabc_B2  Ipu=off  Pbase=100e6  Vbase=Bus(19,2)*1e3  OutputType=Complex  PhasorSimulation=off  PSBequivalent=0
  20 : spsThreePhaseVIMeasurementLib/Three-Phase V-I Measurement  VoltageMeasurement=phase-to-phase  SetLabelV=on  LabelV=Vabc_20  Vpu=off  VpuLL=on  CurrentMeasurement=no  SetLabelI=on  LabelI=Iabc_B2  Ipu=off  Pbase=100e6  Vbase=Bus(20,2)*1e3  OutputType=Complex  PhasorSimulation=off  PSBequivalent=0
  21 : spsThreePhaseVIMeasurementLib/Three-Phase V-I Measurement  VoltageMeasurement=phase-to-phase  SetLabelV=on  LabelV=Vabc_33  Vpu=off  VpuLL=off  CurrentMeasurement=yes  SetLabelI=on  LabelI=Iabc_33  Ipu=off  Pbase=100e6  Vbase=Bus(33,2)*1e3  OutputType=Complex  PhasorSimulation=off  PSBequivalent=0
  22 : spsThreePhaseVIMeasurementLib/Three-Phase V-I Measurement  VoltageMeasurement=phase-to-phase  SetLabelV=on  LabelV=Vabc_22  Vpu=off  VpuLL=on  CurrentMeasurement=no  SetLabelI=on  LabelI=Iabc_B2  Ipu=off  Pbase=100e6  Vbase=Bus(22,2)*1e3  OutputType=Complex  PhasorSimulation=off  PSBequivalent=0
  23 : spsThreePhaseVIMeasurementLib/Three-Phase V-I Measurement  VoltageMeasurement=phase-to-phase  SetLabelV=on  LabelV=Vabc_21  Vpu=off  VpuLL=on  CurrentMeasurement=no  SetLabelI=on  LabelI=Iabc_B2  Ipu=off  Pbase=100e6  Vbase=Bus(21,2)*1e3  OutputType=Complex  PhasorSimulation=off  PSBequivalent=0
  23-1 : spsThreePhaseSeriesRLCBranchLib/Three-Phase Series RLC Branch  LConnTagsString=A|B|C  RConnTagsString=A|B|C  BranchType=RL  Resistance=line(23,3)  Inductance=line(23,4)  Capacitance=1e-6  Measurements=None
  24 : spsThreePhaseVIMeasurementLib/Three-Phase V-I Measurement  VoltageMeasurement=phase-to-phase  SetLabelV=on  LabelV=Vabc_35  Vpu=off  VpuLL=on  CurrentMeasurement=no  SetLabelI=on  LabelI=Iabc_B2  Ipu=off  Pbase=100e6  Vbase=Bus(35,2)*1e3  OutputType=Complex  PhasorSimulation=off  PSBequivalent=0
  24-1 : spsThreePhaseSeriesRLCBranchLib/Three-Phase Series RLC Branch  LConnTagsString=A|B|C  RConnTagsString=A|B|C  BranchType=RL  Resistance=line(24,3)  Inductance=line(24,4)  Capacitance=1e-6  Measurements=None
  26-1 : spsThreePhaseSeriesRLCBranchLib/Three-Phase Series RLC Branch  LConnTagsString=A|B|C  RConnTagsString=A|B|C  BranchType=RL  Resistance=line(26,3)  Inductance=line(26,4)  Capacitance=1e-6  Measurements=None
  27-1 : spsThreePhaseSeriesRLCBranchLib/Three-Phase Series RLC Branch  LConnTagsString=A|B|C  RConnTagsString=A|B|C  BranchType=RL  Resistance=line(27,3)  Inductance=line(27,4)  Capacitance=1e-6  Measurements=None
  28-1 : spsThreePhaseSeriesRLCBranchLib/Three-Phase Series RLC Branch  LConnTagsString=A|B|C  RConnTagsString=A|B|C  BranchType=RL  Resistance=line(28,3)  Inductance=line(28,4)  Capacitance=1e-6  Measurements=None
  33 : spsThreePhaseVIMeasurementLib/Three-Phase V-I Measurement  VoltageMeasurement=phase-to-phase  SetLabelV=on  LabelV=Vabc_24  Vpu=off  VpuLL=on  CurrentMeasurement=no  SetLabelI=on  LabelI=Iabc_B2  Ipu=off  Pbase=100e6  Vbase=Bus(24,2)*1e3  OutputType=Complex  PhasorSimulation=off  PSBequivalent=0
  34 : spsThreePhaseVIMeasurementLib/Three-Phase V-I Measurement  VoltageMeasurement=phase-to-phase  SetLabelV=on  LabelV=Vabc_34  Vpu=off  VpuLL=off  CurrentMeasurement=yes  SetLabelI=on  LabelI=Iabc_34  Ipu=off  Pbase=100e6  Vbase=Bus(34,2)*1e3  OutputType=Complex  PhasorSimulation=off  PSBequivalent=0
  34-1 : spsThreePhaseSeriesRLCBranchLib/Three-Phase Series RLC Branch  LConnTagsString=A|B|C  RConnTagsString=A|B|C  BranchType=RL  Resistance=line(34,3)  Inductance=line(34,4)  Capacitance=1e-6  Measurements=None
  35 : spsThreePhaseVIMeasurementLib/Three-Phase V-I Measurement  VoltageMeasurement=phase-to-phase  SetLabelV=on  LabelV=Vabc_36  Vpu=off  VpuLL=on  CurrentMeasurement=no  SetLabelI=on  LabelI=Iabc_B2  Ipu=off  Pbase=100e6  Vbase=Bus(36,2)*1e3  OutputType=Complex  PhasorSimulation=off  PSBequivalent=0
  35-1 : spsThreePhaseSeriesRLCBranchLib/Three-Phase Series RLC Branch  LConnTagsString=A|B|C  RConnTagsString=A|B|C  BranchType=RL  Resistance=line(35,3)  Inductance=line(35,4)  Capacitance=1e-6  Measurements=None
  36 : spsThreePhaseVIMeasurementLib/Three-Phase V-I Measurement  VoltageMeasurement=phase-to-phase  SetLabelV=on  LabelV=Vabc_23  Vpu=off  VpuLL=on  CurrentMeasurement=no  SetLabelI=on  LabelI=Iabc_B2  Ipu=off  Pbase=100e6  Vbase=Bus(23,2)*1e3  OutputType=Complex  PhasorSimulation=off  PSBequivalent=0
  37-1 : spsThreePhaseSeriesRLCBranchLib/Three-Phase Series RLC Branch  LConnTagsString=A|B|C  RConnTagsString=A|B|C  BranchType=RL  Resistance=line(37,3)  Inductance=line(37,4)  Capacitance=1e-6  Measurements=None
  G4 : Subsystem
  G5(GFL6) : Subsystem  mask{Pnom=Sb, Vnom=Vb(6), Fnom=fb, Vdc_nom=Vdc(6), RLC_Filter=[r_f(6) l_f(6) c_f(6)], Pref=pset(6), Qref=qset(6), PLL_p=kp_pll(6), PLL_i=ki_pll(6), Voltage_P=kp_q(6), Voltage_I=ki_q(6), Current_P=kp_i(6), Current_I=ki_i(6), Power_P=kp_p(6), Power_I=ki_p(6), kf=1, InitialV=Init_GFL(6)}
      mask prompts: Pnom "Rated Power(VA)"; Vnom "Rated L-L RMS Voltage(V)"; Fnom "Rated Frequency(Hz)"; Vdc_nom "DC capacitor voltage(V)"; RLC_Filter "Grid-side coupling impedance(p.u.)"; Pref "Active Power Setting"; Qref "Reactive Power Setting"; PLL_p "PL Proportional Gain"; PLL_i "PLL Integral Gain"; Voltage_P "Voltage Proportional Gain"; Voltage_I "Voltage Integral Gain"; Current_P "Current Proportional Gain"; Current_I "Current Integral Gain"; Power_P "Power Proportional Gain"; Power_I "Power Integral Gain"; kf "Feedforward Gain"; InitialV "Initial Condition"
      mask init:
      | R_f=RLC_Filter(1);
      | L_f=RLC_Filter(2);
      | C_f=RLC_Filter(3);
      mask Display: disp('GFL');
  G6(GFL3) : Subsystem  mask{Pnom=Sb, Vnom=Vb(3), Fnom=fb, Vdc_nom=Vdc(3), RLC_Filter=[r_f(3) l_f(3) c_f(3)], Pref=pset(3), Qref=qset(3), PLL_p=kp_pll(3), PLL_i=ki_pll(3), Voltage_P=kp_q(3), Voltage_I=ki_q(3), Current_P=kp_i(3), Current_I=ki_i(3), Power_P=kp_p(3), Power_I=ki_p(3), kf=1, InitialV=Init_GFL(3)}
      mask prompts: Pnom "Rated Power(VA)"; Vnom "Rated L-L RMS Voltage(V)"; Fnom "Rated Frequency(Hz)"; Vdc_nom "DC capacitor voltage(V)"; RLC_Filter "Grid-side coupling impedance(p.u.)"; Pref "Active Power Setting"; Qref "Reactive Power Setting"; PLL_p "PL Proportional Gain"; PLL_i "PLL Integral Gain"; Voltage_P "Voltage Proportional Gain"; Voltage_I "Voltage Integral Gain"; Current_P "Current Proportional Gain"; Current_I "Current Integral Gain"; Power_P "Power Proportional Gain"; Power_I "Power Integral Gain"; kf "Feedforward Gain"; InitialV "Initial Condition"
      mask init:
      | R_f=RLC_Filter(1);
      | L_f=RLC_Filter(2);
      | C_f=RLC_Filter(3);
      mask Display: disp('GFL');
  G7(GFM2) : Subsystem  mask{Sbnorm=Sb, Vbnorm=Vb_gfm, fbnorm=fb, Vdcnorm=Vdc_gfm(2), RLCnorm=[r_f_gfm(2) l_f_gfm(2) c_f_gfm(2)], P_setnorm=P_set_gfm(2), Q_setnorm=Q_set_gfm(2), Jnorm=J_gfm(2), Dpnorm=D_p_gfm(2), Dqnorm=D_q_gfm(2), Voltage_P=kp_vc_gfm(2), Voltage_I=ki_vc_gfm(2), Current_P=kp_i_gfm(2), Current_I=ki_i_gfm(2), InitialV=Init(2)}
      mask prompts: Sbnorm "Rated Power (VA)"; Vbnorm "Rated L-L RMS Voltage (V)"; fbnorm "Rated frequency (Hz)"; Vdcnorm "DC Voltage (V)"; RLCnorm "Grid-side coupling impedance (real)"; P_setnorm "Power Setting (W)"; Q_setnorm "Reactive Power Setting (W)"; Jnorm "Inertia"; Dpnorm "Power Damping"; Dqnorm "Reactive Power Droop"; Voltage_P "Voltage Proportional Gain"; Voltage_I "Voltage Integral Gain"; Current_P "Current Proportional Gain"; Current_I "Current Integral Gain"; InitialV "Initial Condition"
      mask Display: disp('GFM');
  T2: 900MVA 20 kV/230 kV10 : spsThreePhaseTransformerTwoWindingsLib/Three-Phase Transformer (Two Windings)  Winding1Connection=Delta (D1)  Winding2Connection=Yg  CoreType=Three single-phase transformers  SetSaturation=off  Hysteresis=off  DataFile='hysteresis'  SetInitialFlux=off  Measurements=None  UNITS=pu  NominalPower=[ 100e6 60 ]  Winding1="[ 22e3*1.0   0.00035  0]"  Winding2="[ 345e3*1.0  0.00035  0.0142]"  Rm=500  Lm=500  L0=0.5  Saturation="[ 0,0  ;  0.005,1.2  ;  1.0,1.4 ]"  InitialFluxes=[ 0.8 , -0.8 , 0.7 ]  BreakLoop=off  DiscreteSolver=Trapezoidal iterative  DataType=off  TransfoNumber=0
  T2: 900MVA 20 kV/230 kV11 : spsThreePhaseTransformerTwoWindingsLib/Three-Phase Transformer (Two Windings)  Winding1Connection=Delta (D1)  Winding2Connection=Yg  CoreType=Three single-phase transformers  SetSaturation=off  Hysteresis=off  DataFile='hysteresis'  SetInitialFlux=off  Measurements=None  UNITS=pu  NominalPower=[ 100e6 60 ]  Winding1="[ 22e3*1.0  1e-6  0]"  Winding2="[ 345e3*1.0  1e-6  0.0143]"  Rm=500  Lm=500  L0=0.5  Saturation="[ 0,0  ;  0.005,1.2  ;  1.0,1.4 ]"  InitialFluxes=[ 0.8 , -0.8 , 0.7 ]  BreakLoop=off  DiscreteSolver=Trapezoidal iterative  DataType=off  TransfoNumber=0
  T2: 900MVA 20 kV/230 kV12 : spsThreePhaseTransformerTwoWindingsLib/Three-Phase Transformer (Two Windings)  Winding1Connection=Delta (D1)  Winding2Connection=Yg  CoreType=Three single-phase transformers  SetSaturation=off  Hysteresis=off  DataFile='hysteresis'  SetInitialFlux=off  Measurements=None  UNITS=pu  NominalPower=[ 100e6 60 ]  Winding1="[ 22e3    0.00025  0.0]"  Winding2="[ 345e3    0.00025  0.0272]"  Rm=500  Lm=500  L0=0.5  Saturation="[ 0,0  ;  0.005,1.2  ;  1.0,1.4 ]"  InitialFluxes=[ 0.8 , -0.8 , 0.7 ]  BreakLoop=off  DiscreteSolver=Trapezoidal iterative  DataType=off  TransfoNumber=0
  T2: 900MVA 20 kV/230 kV8 : spsThreePhaseTransformerTwoWindingsLib/Three-Phase Transformer (Two Windings)  Winding1Connection=Y  Winding2Connection=Y  CoreType=Three single-phase transformers  SetSaturation=off  Hysteresis=off  DataFile='hysteresis'  SetInitialFlux=off  Measurements=None  UNITS=pu  NominalPower=[ 100e6 60 ]  Winding1="[ 345e3*1.0  0.00035   0]"  Winding2="[ 345e3*1.00 0.00035  0.0138]"  Rm=500  Lm=500  L0=0.5  Saturation="[ 0,0  ;  0.005,1.2  ;  1.0,1.4 ]"  InitialFluxes=[ 0.8 , -0.8 , 0.7 ]  BreakLoop=off  DiscreteSolver=Trapezoidal iterative  DataType=off  TransfoNumber=0
  T2: 900MVA 20 kV/230 kV9 : spsThreePhaseTransformerTwoWindingsLib/Three-Phase Transformer (Two Windings)  Winding1Connection=Delta (D1)  Winding2Connection=Yg  CoreType=Three single-phase transformers  SetSaturation=off  Hysteresis=off  DataFile='hysteresis'  SetInitialFlux=off  Measurements=None  UNITS=pu  NominalPower=[ 100e6 60 ]  Winding1="[ 22e3*1.00 0.00045  0]"  Winding2="[ 345e3*1  0.00045  0.0180]"  Rm=500  Lm=500  L0=0.5  Saturation="[ 0,0  ;  0.005,1.2  ;  1.0,1.4 ]"  InitialFluxes=[ 0.8 , -0.8 , 0.7 ]  BreakLoop=off  DiscreteSolver=Trapezoidal iterative  DataType=off  TransfoNumber=0
  load15 : spsThreePhaseParallelRLCLoadLib/Three-Phase Parallel RLC Load  LConnTagsString=A|B|C  Configuration=Y (grounded)  NominalVoltage=(345000)*0.969586  Vabc=[1e3 1e3 1e3]  Vabcp=[1e3 1e3 1e3]  NominalFrequency=60  UnbalancedPower=off  ActivePower=320e6  InductivePower=153e6  CapacitivePower=0  Pabc=[10e3 9e3 11e3]  QLabc=[100 90 110]  QCabc=[100 90 110]  Pabcp=[10e3 9e3 11e3]  QLabcp=[100 90 110]  QCabcp=[100 90 110]  Measurements=None  LoadType=constant PQ
  load16 : spsThreePhaseParallelRLCLoadLib/Three-Phase Parallel RLC Load  LConnTagsString=A|B|C  Configuration=Y (grounded)  NominalVoltage=(345000)*0.988678  Vabc=[1e3 1e3 1e3]  Vabcp=[1e3 1e3 1e3]  NominalFrequency=60  UnbalancedPower=off  ActivePower=329e6  InductivePower=32.3e6  CapacitivePower=0  Pabc=[10e3 9e3 11e3]  QLabc=[100 90 110]  QCabc=[100 90 110]  Pabcp=[10e3 9e3 11e3]  QLabcp=[100 90 110]  QCabcp=[100 90 110]  Measurements=None  LoadType=constant PQ
  load20 : spsThreePhaseParallelRLCLoadLib/Three-Phase Parallel RLC Load  LConnTagsString=A|B|C  Configuration=Y (grounded)  NominalVoltage=(345000)*0.987086  Vabc=[1e3 1e3 1e3]  Vabcp=[1e3 1e3 1e3]  NominalFrequency=60  UnbalancedPower=off  ActivePower=628e6  InductivePower=103e6  CapacitivePower=0  Pabc=[10e3 9e3 11e3]  QLabc=[100 90 110]  QCabc=[100 90 110]  Pabcp=[10e3 9e3 11e3]  QLabcp=[100 90 110]  QCabcp=[100 90 110]  Measurements=None  LoadType=constant PQ
  load21 : spsThreePhaseParallelRLCLoadLib/Three-Phase Parallel RLC Load  LConnTagsString=A|B|C  Configuration=Y (grounded)  NominalVoltage=(345000)*0.995503  Vabc=[1e3 1e3 1e3]  Vabcp=[1e3 1e3 1e3]  NominalFrequency=60  UnbalancedPower=off  ActivePower=274e6  InductivePower=115e6  CapacitivePower=0  Pabc=[10e3 9e3 11e3]  QLabc=[100 90 110]  QCabc=[100 90 110]  Pabcp=[10e3 9e3 11e3]  QLabcp=[100 90 110]  QCabcp=[100 90 110]  Measurements=None  LoadType=constant PQ
  load23 : spsThreePhaseParallelRLCLoadLib/Three-Phase Parallel RLC Load  LConnTagsString=A|B|C  Configuration=Y (grounded)  NominalVoltage=(345000)*1.02041  Vabc=[1e3 1e3 1e3]  Vabcp=[1e3 1e3 1e3]  NominalFrequency=60  UnbalancedPower=off  ActivePower=247.5e6  InductivePower=84.6e6  CapacitivePower=0  Pabc=[10e3 9e3 11e3]  QLabc=[100 90 110]  QCabc=[100 90 110]  Pabcp=[10e3 9e3 11e3]  QLabcp=[100 90 110]  QCabcp=[100 90 110]  Measurements=None  LoadType=constant PQ
  load24 : spsThreePhaseParallelRLCLoadLib/Three-Phase Parallel RLC Load  LConnTagsString=A|B|C  Configuration=Y (grounded)  NominalVoltage=(345000)*0.996934  Vabc=[1e3 1e3 1e3]  Vabcp=[1e3 1e3 1e3]  NominalFrequency=60  UnbalancedPower=off  ActivePower=308.6e6  InductivePower=0  CapacitivePower=92.2e6  Pabc=[10e3 9e3 11e3]  QLabc=[100 90 110]  QCabc=[100 90 110]  Pabcp=[10e3 9e3 11e3]  QLabcp=[100 90 110]  QCabcp=[100 90 110]  Measurements=None  LoadType=constant PQ
  C : PMIOPort  Side=Left
  B : PMIOPort  Port=2  Side=Left
  A : PMIOPort  Port=3  Side=Left
  a : PMIOPort  Port=4  Side=Right
  b : PMIOPort  Port=5  Side=Right
  c : PMIOPort  Port=6  Side=Right
  tag scope: Pe5=global, Pe6=global, Pe7=global, Q5=global, Q6=global, Q7=global, U5=global, U6=global, U7=global, theta05=global, theta06=global, theta07=global, theta5=global, theta6=global, theta7=global, w5=global, w6=global, w7=global
  wires:
  G6(GFL3)/1(P) -> [Pe6]
  G6(GFL3)/2(Omega) -> [w6]
  G6(GFL3)/3(Vabs) -> [U6]
  G6(GFL3)/4(theta_t) -> [theta6]
  G6(GFL3)/5(Q) -> [Q6]
  G6(GFL3)/6(theta_0) -> [theta06]
  G7(GFM2)/1(P) -> [Pe7]
  G7(GFM2)/2(Omega) -> [w7]
  G7(GFM2)/3(Vabs) -> [U7]
  G7(GFM2)/4(theta_t) -> [theta7]
  G7(GFM2)/5(theta_0) -> [theta07]
  G7(GFM2)/6(Q) -> [Q7]
  G5(GFL6)/3(Vabs) -> [U5]
  G5(GFL6)/2(Omega) -> [w5]
  G5(GFL6)/1(P) -> [Pe5]
  G5(GFL6)/4(theta_t) -> [theta5]
  G5(GFL6)/6(theta_0) -> [theta05]
  G5(GFL6)/5(Q) -> [Q5]
  connections:
  T2: 900MVA 20 kV/230 kV10/LConn1 -- 21/RConn1
  23-1/LConn2 -- 15/RConn2 -- load15/LConn2
  load20/LConn1 -- T2: 900MVA 20 kV/230 kV9/RConn1 -- 20/RConn1
  T2: 900MVA 20 kV/230 kV12/LConn2 -- 35/LConn2
  24-1/LConn1 -- 16/LConn1 -- 26-1/LConn1 -- 27-1/RConn1
  T2: 900MVA 20 kV/230 kV12/LConn3 -- 35/LConn3
  T2: 900MVA 20 kV/230 kV11/RConn2 -- 35-1/LConn2 -- 22/RConn2
  T2: 900MVA 20 kV/230 kV8/LConn3 -- 19/RConn3
  26-1/RConn1 -- 19/LConn1 -- T2: 900MVA 20 kV/230 kV10/RConn1
  36/LConn1 -- 37-1/RConn1 -- 35-1/RConn1
  23-1/LConn1 -- load15/LConn1 -- 15/RConn1
  T2: 900MVA 20 kV/230 kV8/RConn2 -- 20/LConn2
  load23/LConn2 -- 36/RConn2 -- T2: 900MVA 20 kV/230 kV12/RConn2
  37-1/LConn1 -- load24/LConn1 -- 33/RConn1
  24-1/LConn2 -- 26-1/LConn2 -- 27-1/RConn2 -- 16/LConn2
  load21/LConn1 -- 34-1/LConn1 -- 23/RConn1
  35-1/LConn1 -- 22/RConn1 -- T2: 900MVA 20 kV/230 kV11/RConn1
  load16/LConn3 -- C/RConn1 -- 28-1/RConn3 -- 16/RConn3
  36/LConn3 -- 37-1/RConn3 -- 35-1/RConn3
  T2: 900MVA 20 kV/230 kV8/RConn1 -- 20/LConn1
  37-1/LConn3 -- load24/LConn3 -- 33/RConn3
  26-1/RConn3 -- T2: 900MVA 20 kV/230 kV10/RConn3 -- 19/LConn3
  T2: 900MVA 20 kV/230 kV12/LConn1 -- 35/LConn1
  23-1/LConn3 -- 15/RConn3 -- load15/LConn3
  37-1/LConn2 -- load24/LConn2 -- 33/RConn2
  36/LConn2 -- 37-1/RConn2 -- 35-1/RConn2
  T2: 900MVA 20 kV/230 kV11/LConn3 -- 24/LConn3
  23-1/RConn2 -- b/RConn1
  T2: 900MVA 20 kV/230 kV8/LConn2 -- 19/RConn2
  T2: 900MVA 20 kV/230 kV9/LConn3 -- 34/LConn3
  16/LConn3 -- 26-1/LConn3 -- 27-1/RConn3 -- 24-1/LConn3
  load23/LConn1 -- T2: 900MVA 20 kV/230 kV12/RConn1 -- 36/RConn1
  23/RConn2 -- 34-1/LConn2 -- load21/LConn2
  28-1/LConn2 -- 33/LConn2
  28-1/LConn3 -- 33/LConn3
  28-1/LConn1 -- 33/LConn1
  T2: 900MVA 20 kV/230 kV11/LConn2 -- 24/LConn2
  27-1/LConn2 -- 23/LConn2
  T2: 900MVA 20 kV/230 kV11/RConn3 -- 35-1/LConn3 -- 22/RConn3
  16/RConn1 -- A/RConn1 -- 28-1/RConn1 -- load16/LConn1
  16/RConn2 -- B/RConn1 -- 28-1/RConn2 -- load16/LConn2
  T2: 900MVA 20 kV/230 kV10/LConn3 -- 21/RConn3
  load20/LConn3 -- T2: 900MVA 20 kV/230 kV9/RConn3 -- 20/RConn3
  27-1/LConn3 -- 23/LConn3
  27-1/LConn1 -- 23/LConn1
  26-1/RConn2 -- 19/LConn2 -- T2: 900MVA 20 kV/230 kV10/RConn2
  load23/LConn3 -- T2: 900MVA 20 kV/230 kV12/RConn3 -- 36/RConn3
  24-1/RConn1 -- 15/LConn1
  24-1/RConn3 -- 15/LConn3
  24-1/RConn2 -- 15/LConn2
  T2: 900MVA 20 kV/230 kV8/LConn1 -- 19/RConn1
  23/RConn3 -- 34-1/LConn3 -- load21/LConn3
  load20/LConn2 -- T2: 900MVA 20 kV/230 kV9/RConn2 -- 20/RConn2
  T2: 900MVA 20 kV/230 kV9/LConn2 -- 34/LConn2
  T2: 900MVA 20 kV/230 kV9/LConn1 -- 34/LConn1
  T2: 900MVA 20 kV/230 kV11/LConn1 -- 24/LConn1
  T2: 900MVA 20 kV/230 kV8/RConn3 -- 20/LConn3
  T2: 900MVA 20 kV/230 kV10/LConn2 -- 21/RConn2
  23-1/RConn1 -- a/RConn1
  23-1/RConn3 -- c/RConn1
  G7(GFM2)/RConn1 -- 35/RConn1
  G7(GFM2)/RConn2 -- 35/RConn2
  G7(GFM2)/RConn3 -- 35/RConn3
  24/RConn1 -- G6(GFL3)/RConn1
  24/RConn2 -- G6(GFL3)/RConn2
  24/RConn3 -- G6(GFL3)/RConn3
  G4/RConn1 -- 21/LConn1
  G4/RConn2 -- 21/LConn2
  G4/RConn3 -- 21/LConn3
  22/LConn1 -- 34-1/RConn1
  22/LConn2 -- 34-1/RConn2
  22/LConn3 -- 34-1/RConn3
  G5(GFL6)/RConn1 -- 34/RConn1
  G5(GFL6)/RConn2 -- 34/RConn2
  G5(GFL6)/RConn3 -- 34/RConn3

== system IEEE_39_case2/Measure ==
  W_gens{,1..3} (4 alike) : Mux  Inputs=10
  w : Outport  VectorParamsAs1DForOutWhenUnconnected=off
  Pe : Outport  Port=2
  U : Outport  Port=3
  Q : Outport  Port=4
  wires:
  W_gens/1 -> w/1  "w"
  [w1] -> W_gens/1
  [w2] -> W_gens/2
  [w4] -> W_gens/4
  [w3] -> W_gens/3
  [w5] -> W_gens/5
  [w9] -> W_gens/9
  [w8] -> W_gens/8
  [w7] -> W_gens/7
  [w6] -> W_gens/6
  [w10] -> W_gens/10
  [Pe6] -> W_gens1/6
  [Pe3] -> W_gens1/3
  [Pe7] -> W_gens1/7
  [Pe5] -> W_gens1/5
  [Pe9] -> W_gens1/9
  [U5] -> W_gens2/5
  [U3] -> W_gens2/3
  [Pe1] -> W_gens1/1
  [Pe4] -> W_gens1/4
  [U9] -> W_gens2/9
  [U7] -> W_gens2/7
  [U8] -> W_gens2/8
  [U6] -> W_gens2/6
  [U1] -> W_gens2/1
  [Pe2] -> W_gens1/2
  [U2] -> W_gens2/2
  [U10] -> W_gens2/10
  W_gens1/1 -> Pe/1
  [U4] -> W_gens2/4
  W_gens2/1 -> U/1
  [Pe10] -> W_gens1/10
  [Pe8] -> W_gens1/8
  [Q2] -> W_gens3/2
  [Q1] -> W_gens3/1
  W_gens3/1 -> Q/1
  [Q3] -> W_gens3/3
  [Q10] -> W_gens3/10
  [Q6] -> W_gens3/6
  [Q7] -> W_gens3/7
  [Q4] -> W_gens3/4
  [Q5] -> W_gens3/5
  [Q8] -> W_gens3/8
  [Q9] -> W_gens3/9
